simulink model "schem_3"  (R2024a)
settings: Solver=FixedStepAuto  StartTime=0.0  StopTime=10.0  FixedStep=0.2  RelTol=1e-3
undefined symbols (not defined in the file): T_d_z0, T_d_z1, T_d_z2, T_d_z3, T_n_z0, T_n_z1, T_n_z2, T_n_z3
settings Model: Creator=user  LastModifiedBy=user

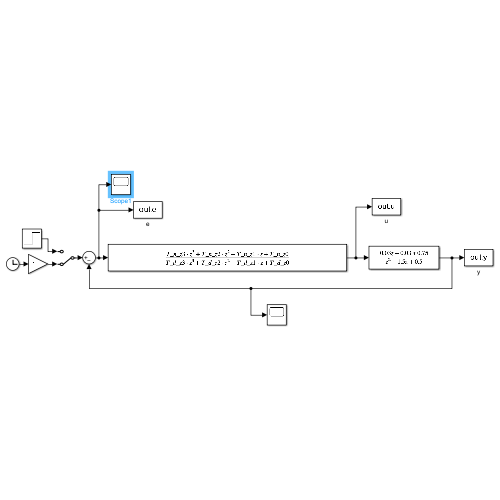
[thumbnail: Simulink's stored preview of the top-level diagram]
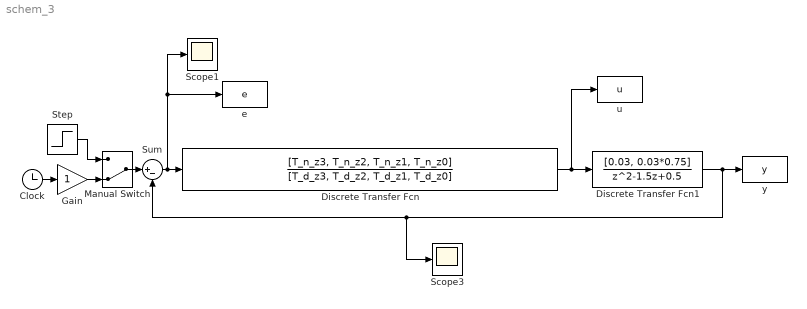
== system schem_3 ==
  Clock : Clock
  Discrete Transfer Fcn : DiscreteTransferFcn  Numerator=[T_n_z3, T_n_z2, T_n_z1, T_n_z0]  Denominator=[T_d_z3, T_d_z2, T_d_z1, T_d_z0]
  Discrete Transfer Fcn1 : DiscreteTransferFcn  Numerator=[0.03, 0.03*0.75]  Denominator=[1, -1.5, 0.5]
  Gain : Gain
  Manual Switch : ManualSwitch  CurrentSetting=0
  Scope1 : Scope
  Scope3 : Scope
  Step : Step  SampleTime=0
  Sum : Sum  Inputs=|+-
  e : ToWorkspace  VariableName=e  SaveFormat=Timeseries  SampleTime=-1
  u : ToWorkspace  VariableName=u  SaveFormat=Timeseries  SampleTime=-1
  y : ToWorkspace  VariableName=y  SaveFormat=Timeseries  SampleTime=-1
  wires:
  Discrete Transfer Fcn/1 -> u/1, Discrete Transfer Fcn1/1
  Discrete Transfer Fcn1/1 -> Scope3/1, Sum/2, y/1
  Sum/1 -> Scope1/1, e/1, Discrete Transfer Fcn/1
  Clock/1 -> Gain/1
  Step/1 -> Manual Switch/1
  Manual Switch/1 -> Sum/1
  Gain/1 -> Manual Switch/2
